simulink model "Rotor_drivetrain"  (R2018b)
settings: Solver=VariableStepAuto  StartTime=0.0  StopTime=10.0  RelTol=1e-3
libraries: fmu_me_lib x1
settings Model: Creator=Bob  LastModifiedBy=meagh
settings DataIOCC: ReturnWorkspaceOutputs=on
settings RTWCC: SystemTargetFile=fmu_me1.tlc  MakeCommand=make_rtw FMIT_INTERMEDIATE_LIB_DIR=DEFAULT  TemplateMakefile=fmu_me1_default_tmf  Description=FMU Model Exchange 1.0
settings STFCustomTargetCC: TargetLangStandard=C99 (ISO)  ModelReferenceCompliant=off  MATLABClassNameForMDSCustomization=Simulink.SoftwareTarget.TargetSpecificTriggerConfigurationBase  GRTInterface=on  SystemTargetFile=fmu_me1.tlc

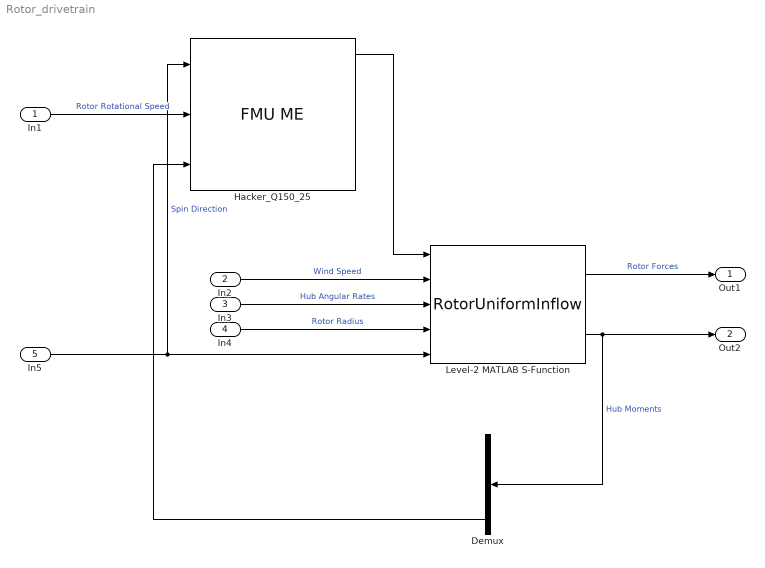
== system Rotor_drivetrain ==
  In1 : Inport  OutDataTypeStr=double
  In2 : Inport  Port=2  OutDataTypeStr=double
  In3 : Inport  Port=3  OutDataTypeStr=double
  In4 : Inport  Port=4  OutDataTypeStr=double
  In5 : Inport  Port=5  OutDataTypeStr=boolean
  Demux : Demux  Outputs=3
  Hacker_Q150_25 : fmu_me_lib/FMU ME  Description=Simulates an FMU for Model Exchange 1.0 or Model Exchange 2.0.  dummy=0
  Level-2 MATLAB S-Function : M-S-Function  FunctionName=RotorUniformInflow
  Out1 : Outport  OutDataTypeStr=double
  Out2 : Outport  Port=2  OutDataTypeStr=double
  wires:
  Level-2 MATLAB S-Function/1 -> Out1/1  "Rotor Forces"
  Level-2 MATLAB S-Function/2 -> Demux/1, Out2/1  "Hub Moments"
  In4/1 -> Level-2 MATLAB S-Function/4  "Rotor Radius"
  In2/1 -> Level-2 MATLAB S-Function/2  "Wind Speed"
  In1/1 -> Hacker_Q150_25/2  "Rotor Rotational Speed"
  In5/1 -> Hacker_Q150_25/1, Level-2 MATLAB S-Function/5  "Spin Direction"
  Hacker_Q150_25/1 -> Level-2 MATLAB S-Function/1
  In3/1 -> Level-2 MATLAB S-Function/3  "Hub Angular Rates"
  Demux/3 -> Hacker_Q150_25/3
